simulink model "sim"  (R2017a)
settings: Solver=VariableStepAuto  StartTime=0.0  StopTime=10.0  RelTol=1e-3
libraries: legoev3lib x5, simulink x1
settings Model: Creator=Master  LastModifiedBy=Master

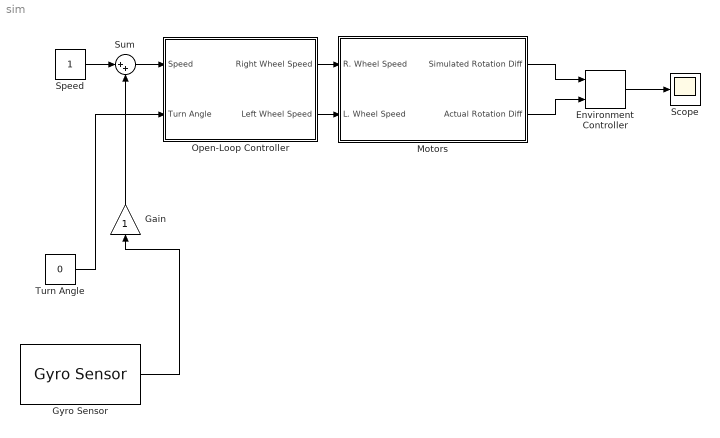
== system sim ==
  Environment Controller : simulink/Signal Routing/Environment Controller
      settings: SourceProductName=Simulink  SourceProductBaseCode=SL
  Gain : Gain
  Gyro Sensor : legoev3lib/Gyro Sensor  portNumber=1  sampleTime=0.1
      settings: SourceProductName=Simulink Support Package for LEGO MINDSTORMS EV3 Hardware  SourceProductBaseCode=LEGOEV3
  Motors : Subsystem  VariantControl=DoSim
  Open-Loop Controller : Subsystem
  Scope : Scope
  Speed : Constant  OutDataTypeStr=single  SampleTime=0.01
  Sum : Sum  Inputs=|++
  Turn Angle : Constant  Value=0  OutDataTypeStr=single  SampleTime=0.01
  wires:
  Sum/1 -> Open-Loop Controller/1(Speed)
  Gain/1 -> Sum/2
  Gyro Sensor/1 -> Gain/1
  Open-Loop Controller/1(Right Wheel Speed) -> Motors/1(R. Wheel Speed)
  Motors/1(Simulated Rotation Diff) -> Environment Controller/1
  Open-Loop Controller/2(Left Wheel Speed) -> Motors/2(L. Wheel Speed)
  Turn Angle/1 -> Open-Loop Controller/2(Turn Angle)
  Motors/2(Actual Rotation Diff) -> Environment Controller/2
  Speed/1 -> Sum/1
  Environment Controller/1 -> Scope/1

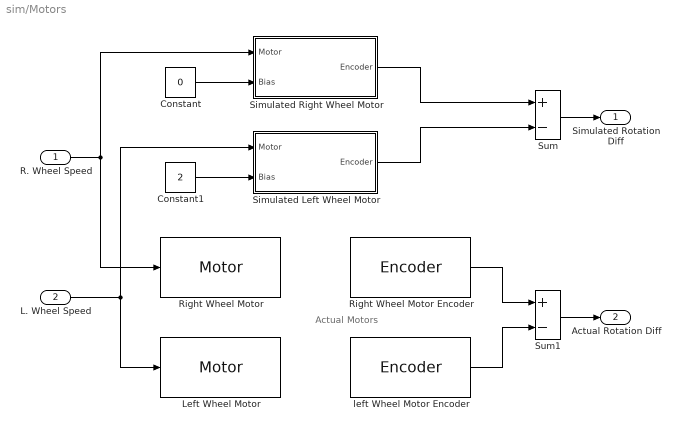
== system sim/Motors ==
  note: Actual
      | Motors
  R. Wheel Speed : Inport
  L. Wheel Speed : Inport  Port=2
  Constant : Constant  Value=0  OutDataTypeStr=single
  Constant1 : Constant  Value=2  OutDataTypeStr=single
  Left Wheel Motor : legoev3lib/Motor  sportNumber=A  sstopAction=Brake
  Right Wheel Motor : legoev3lib/Motor  sportNumber=D  sstopAction=Brake
  Right Wheel Motor Encoder : legoev3lib/Encoder  portNumber=D  opMode=Reset at each sample time  sampleTime=0.1
      settings: SourceProductName=Simulink Support Package for LEGO MINDSTORMS EV3 Hardware  SourceProductBaseCode=LEGOEV3
  Simulated Left Wheel Motor : Subsystem
  Simulated Right Wheel Motor : Subsystem
  Sum : Sum  Inputs=+-  OutDataTypeStr=Inherit: Same as first input
  Sum1 : Sum  Inputs=+-  OutDataTypeStr=Inherit: Same as first input
  left Wheel Motor Encoder : legoev3lib/Encoder  portNumber=A  opMode=Reset at each sample time  sampleTime=0.1
      settings: SourceProductName=Simulink Support Package for LEGO MINDSTORMS EV3 Hardware  SourceProductBaseCode=LEGOEV3
  Simulated Rotation Diff : Outport
  Actual Rotation Diff : Outport  Port=2
  wires:
  Sum1/1 -> Actual Rotation Diff/1
  left Wheel Motor Encoder/1 -> Sum1/2
  Right Wheel Motor Encoder/1 -> Sum1/1
  Sum/1 -> Simulated Rotation Diff/1
  Simulated Left Wheel Motor/1(Encoder) -> Sum/2
  Simulated Right Wheel Motor/1(Encoder) -> Sum/1
  R. Wheel Speed/1 -> Right Wheel Motor/1, Simulated Right Wheel Motor/1(Motor)
  L. Wheel Speed/1 -> Left Wheel Motor/1, Simulated Left Wheel Motor/1(Motor)
  Constant/1 -> Simulated Right Wheel Motor/2(Bias)
  Constant1/1 -> Simulated Left Wheel Motor/2(Bias)

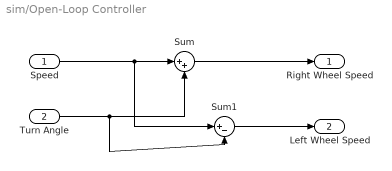
== system sim/Open-Loop Controller ==
  Speed : Inport
  Turn Angle : Inport  Port=2
  Sum : Sum  Inputs=|++  OutDataTypeStr=Inherit: Same as first input
  Sum1 : Sum  Inputs=|+-  OutDataTypeStr=Inherit: Same as first input
  Right Wheel Speed : Outport
  Left Wheel Speed : Outport  Port=2
  wires:
  Sum1/1 -> Left Wheel Speed/1
  Sum/1 -> Right Wheel Speed/1
  Turn Angle/1 -> Sum1/2, Sum/2
  Speed/1 -> Sum1/1, Sum/1

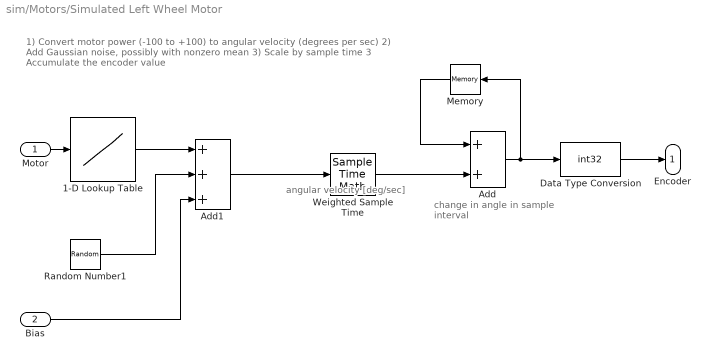
== system sim/Motors/Simulated Left Wheel Motor ==
  note: change in angle
      | in sample interval
  note: angular velocity
      | [deg/sec]
  note: 1) Convert motor power (-100 to +100) to angular velocity (degrees per sec)
      | 2) Add Gaussian noise, possibly with nonzero mean
      | 3) Scale by sample time
      | 3 Accumulate the encoder value
  Motor : Inport
  Bias : Inport  Port=2
  1-D Lookup Table : Lookup_n-D  NumberOfTableDimensions=1  BreakpointsForDimension1=[-100 0 100]  Table=[-360 0 360]  ExtrapMethod=Clip  UseLastTableValue=on  RndMeth=Simplest  InputSameDT=on
  Add : Sum  OutDataTypeStr=Inherit: Same as first input
  Add1 : Sum  Inputs=+++  OutDataTypeStr=single
  Data Type Conversion : DataTypeConversion  OutDataTypeStr=int32
  Memory : Memory  InheritSampleTime=on  LinearizeAsDelay=on
  Random Number1 : RandomNumber  Variance=5  Seed=randi(1000)
  Weighted Sample Time : SampleTimeMath  TsampMathOp=*
  Encoder : Outport
  wires:
  Data Type Conversion/1 -> Encoder/1
  Bias/1 -> Add1/3
  Weighted Sample Time/1 -> Add/2
  Add/1 -> Data Type Conversion/1, Memory/1
  Memory/1 -> Add/1
  Add1/1 -> Weighted Sample Time/1
  Motor/1 -> 1-D Lookup Table/1
  Random Number1/1 -> Add1/2
  1-D Lookup Table/1 -> Add1/1

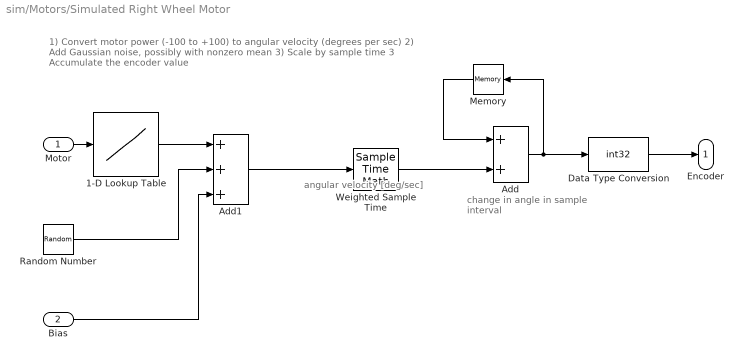
== system sim/Motors/Simulated Right Wheel Motor ==
  note: 1) Convert motor power (-100 to +100) to angular velocity (degrees per sec)
      | 2) Add Gaussian noise, possibly with nonzero mean
      | 3) Scale by sample time
      | 3 Accumulate the encoder value
  note: angular velocity
      |  [deg/sec]
  note: change in angle
      | in sample interval
  Motor : Inport
  Bias : Inport  Port=2
  1-D Lookup Table : Lookup_n-D  NumberOfTableDimensions=1  BreakpointsForDimension1=[-100 0 100]  Table=[-360 0 360]  ExtrapMethod=Clip  UseLastTableValue=on  RndMeth=Simplest  InputSameDT=on
  Add : Sum  AccumDataTypeStr=single  OutDataTypeStr=single
  Add1 : Sum  Inputs=+++  OutDataTypeStr=single
  Data Type Conversion : DataTypeConversion  OutDataTypeStr=int32
  Memory : Memory  InheritSampleTime=on  LinearizeAsDelay=on
  Random Number : RandomNumber  Variance=5  Seed=randi(1000)
  Weighted Sample Time : SampleTimeMath  TsampMathOp=*
  Encoder : Outport
  wires:
  Data Type Conversion/1 -> Encoder/1
  1-D Lookup Table/1 -> Add1/1
  Random Number/1 -> Add1/2
  Motor/1 -> 1-D Lookup Table/1
  Memory/1 -> Add/1
  Add/1 -> Data Type Conversion/1, Memory/1
  Weighted Sample Time/1 -> Add/2
  Bias/1 -> Add1/3
  Add1/1 -> Weighted Sample Time/1
